simulink model "Gear"  (R2023b)
settings: Solver=VariableStepAuto  StartTime=0.0  StopTime=10.0  RelTol=1e-3
values from neighbouring files (symbols this model uses):
  b = 0.1    [paras_Gear.m]
  Capacity = 5    [paras_Gear.m]
  G_ratio = 10    [paras_Gear.m]
  J = 0.01    [paras_Gear.m]
  L = 0.5    [paras_Gear.m]
  R = 1    [paras_Gear.m]
  R_bat = 0.5    [paras_Gear.m]
settings Model: Creator=mdhel  LastModifiedBy=mdhel

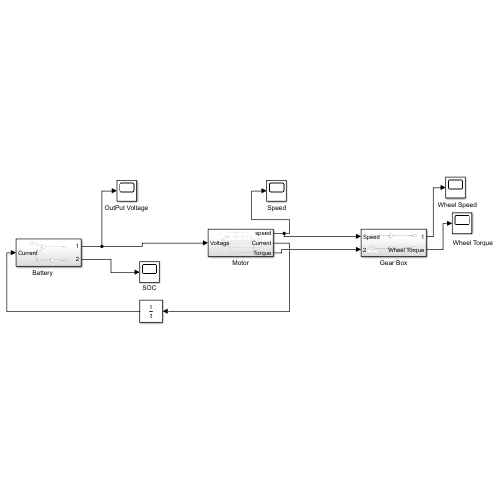
[thumbnail: Simulink's stored preview of the top-level diagram]
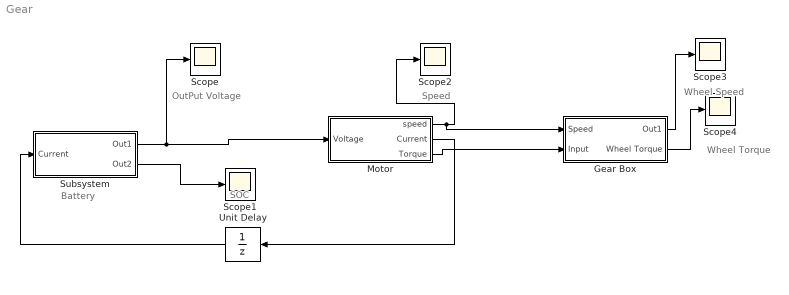
== system Gear ==
  note: Wheel Torque
  note: Wheel Speed
  note: Battery
  note: OutPut Voltage
  note: Speed
  note: SOC
  Gear Box : Subsystem
  Motor : Subsystem
  Scope{,1..4} (5 alike) : Scope
  Subsystem : Subsystem
  Unit Delay : UnitDelay  SampleTime=-1  HasFrameUpgradeWarning=on
  wires:
  Subsystem/2(Out2) -> Scope1/1
  Motor/2(Current) -> Unit Delay/1
  Subsystem/1(Out1) -> Motor/1(Voltage), Scope/1
  Motor/1(speed) -> Gear Box/1(Speed), Scope2/1
  Unit Delay/1 -> Subsystem/1(Current)
  Motor/3(Torque) -> Gear Box/2(Input)
  Gear Box/1(Out1) -> Scope3/1
  Gear Box/2(Wheel Torque) -> Scope4/1

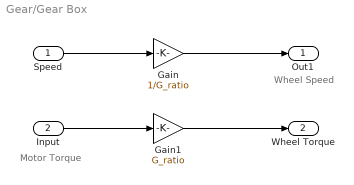
== system Gear/Gear Box ==
  note: Motor Torque
  note: Wheel Speed
  Speed : Inport
  Input : Inport  Port=2
  Gain : Gain  Gain=1/G_ratio
  Gain1 : Gain  Gain=G_ratio
  Out1 : Outport
  Wheel Torque : Outport  Port=2
  wires:
  Speed/1 -> Gain/1
  Gain/1 -> Out1/1
  Input/1 -> Gain1/1
  Gain1/1 -> Wheel Torque/1

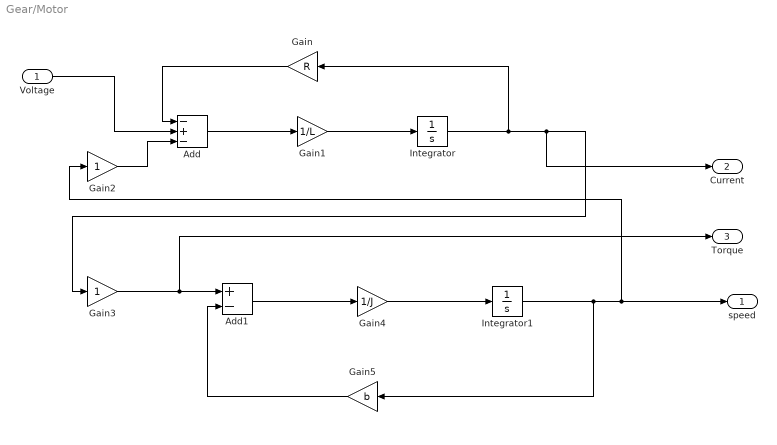
== system Gear/Motor ==
  Voltage : Inport
  Add : Sum  Inputs=-+-
  Add1 : Sum  Inputs=+-
  Gain : Gain  Gain=R
  Gain1 : Gain  Gain=1/L
  Gain2 : Gain
  Gain3 : Gain
  Gain4 : Gain  Gain=1/J
  Gain5 : Gain  Gain=b
  Integrator : Integrator
  Integrator1 : Integrator
  speed : Outport
  Current : Outport  Port=2
  Torque : Outport  Port=3
  wires:
  Voltage/1 -> Add/2
  Gain/1 -> Add/1
  Add/1 -> Gain1/1
  Gain1/1 -> Integrator/1
  Integrator/1 -> Gain/1, Current/1, Gain3/1
  Gain2/1 -> Add/3
  Gain3/1 -> Torque/1, Add1/1
  Add1/1 -> Gain4/1
  Gain4/1 -> Integrator1/1
  Integrator1/1 -> Gain5/1, Gain2/1, speed/1
  Gain5/1 -> Add1/2

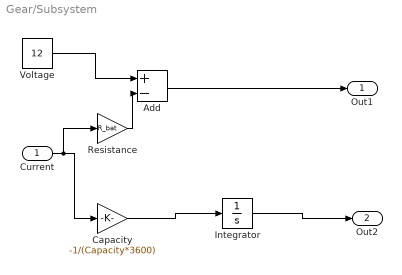
== system Gear/Subsystem ==
  Current : Inport
  Add : Sum  Inputs=+-
  Capacity : Gain  Gain=-1/(Capacity*3600)
  Integrator : Integrator  InitialCondition=1
  Resistance : Gain  Gain=R_bat
  Voltage : Constant  Value=12
  Out1 : Outport
  Out2 : Outport  Port=2
  wires:
  Voltage/1 -> Add/1
  Add/1 -> Out1/1
  Capacity/1 -> Integrator/1
  Integrator/1 -> Out2/1
  Current/1 -> Resistance/1, Capacity/1
  Resistance/1 -> Add/2
